simulink model "sim_switch_vol_hover_rotation"  (R2020b)
settings: Solver=VariableStepAuto  StartTime=0.0  StopTime=T  MaxStep=MaxStep  RelTol=RelTol
values from neighbouring files (symbols this model uses):
  J = drone.INERTIA    [utComputeTrimFlight_fmin_dyn.m]
  T = drone.MASS*drone.G    [utComputeTrimFlight_fmin_dyn.m]
undefined symbols (not defined in the file or in its folder): a, b, controlleur, drone, f_initial, K_complet, K_lin_control, q_d_initial, rule, S_complet, u_eq_hover, u_eq_vol, x0, x_eq_hover, x_eq_vol
libraries: simulink x3, simulink_extras x3, sharedtransform x1
settings Model: Creator=florian  LastModifiedBy=florian

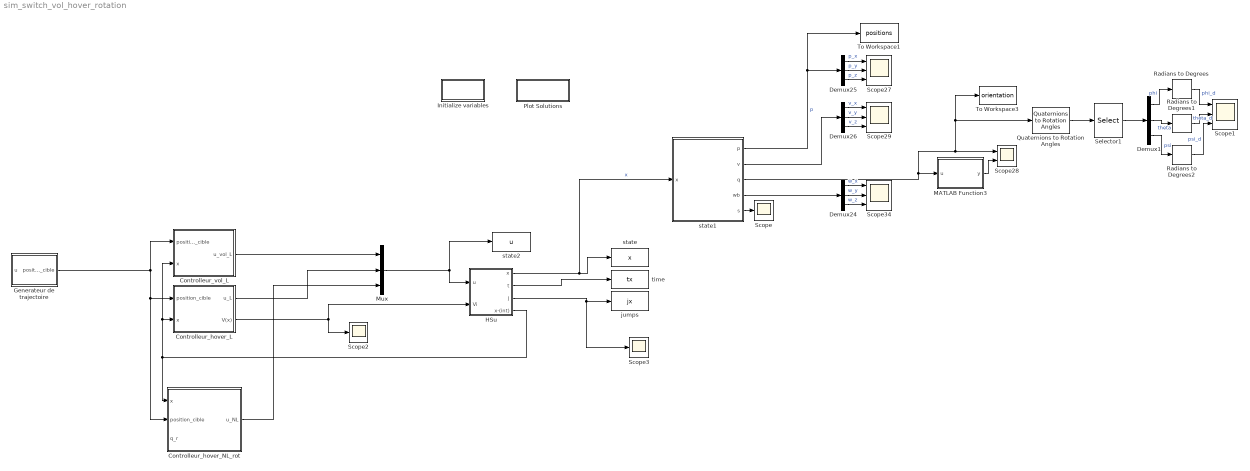
== system sim_switch_vol_hover_rotation ==
  Controlleur_hover_L : Subsystem
  Controlleur_hover_NL_rot : Subsystem
  Controlleur_vol_L : Subsystem
  Demux{1,24..26} (4 alike) : Demux  Outputs=3
  Generateur de trajectoire : MATLAB Function  TreatAsAtomicUnit=on
  HSu : Subsystem  LoadFcn=set_param(gcb,'LinkStatus','none')
      settings: CopyFcn=|
      | set_param(gcb,'LinkStatus','none'),
      | set_param(gcs, 'MaxStep', 'MaxStep', 'RelTol', 'RelTol','Stop time', 'T')
      mask Display:
      | image(imread('Hcal.jpg'))
      | %plot([5 20 20 5 5],[5 5 20 20 5])
      | %text(8,13,'HyEq_mdl')
      | port_label('output', 1, 'x')
      | port_label('output', 2, 't')
      | port_label('output', 3, 'j')
      | port_label('output', 4, 'x-(int)')
      | port_label('input', 1, 'u')
      | port_label('input', 2, 'V(x)')
  Initialize variables : Subsystem  Priority=-10
      settings: OpenFcn=initialization_di
      mask Display: disp('Double Click\n to Initialize')
  MATLAB Function3 : MATLAB Function  TreatAsAtomicUnit=on
  Mux : Mux  Inputs=3
  Plot Solutions : Subsystem
      settings: OpenFcn=postprocessing_di
      mask Display: disp('Double Click to\n Plot Solutions')
  Quaternions to Rotation Angles : sharedtransform/Quaternions to Rotation Angles  rotationOrder=ZXY  aMode=aMode
      settings: SourceProductBaseCode=AE,PW,MT,UV,VE,VP
  Radians to Degrees : simulink_extras/Transformations/Radians to Degrees
  Radians to Degrees1 : simulink_extras/Transformations/Radians to Degrees
  Radians to Degrees2 : simulink_extras/Transformations/Radians to Degrees
  Scope : Scope
  Scope{1,27,29,34} (4 alike) : Scope  NumInputPorts=3
  Scope2 : Scope
  Scope28 : Scope  NumInputPorts=2
  Scope3 : Scope
  Selector1 : Selector  InputPortWidth=3  IndexOptions=Index vector (dialog)  Indices=[2 3 1]  OutputSizes=1
  To Workspace1 : ToWorkspace  VariableName=positions  SampleTime=-1
  To Workspace3 : ToWorkspace  VariableName=orientation  SampleTime=-1
  jumps : ToWorkspace  VariableName=jx  SampleTime=-1
  state : ToWorkspace  VariableName=x  SampleTime=-1
  state1 : MATLAB Function  TreatAsAtomicUnit=on
  state2 : ToWorkspace  VariableName=u  SampleTime=-1
  time : ToWorkspace  VariableName=tx  SampleTime=-1
  wires:
  Mux/1 -> HSu/1(u), state2/1
  HSu/1(x) -> state1/1(x), state/1  "x"
  HSu/2(t) -> time/1
  HSu/3(j) -> jumps/1, Scope3/1
  Controlleur_hover_L/1(u_L) -> Mux/2
  Generateur de trajectoire/1(position_cible) -> Controlleur_vol_L/1(position_cible), Controlleur_hover_NL_rot/2(position_cible), Controlleur_hover_L/1(position_cible)
  Controlleur_hover_L/2(V(x)) -> Scope2/1, HSu/2(Vi)
  HSu/4(x-(int)) -> Controlleur_hover_NL_rot/1(x), Controlleur_vol_L/2(x), Controlleur_hover_L/2(x)
  Demux1/2 -> Radians to Degrees1/1  "theta"
  Quaternions to Rotation Angles/1 -> Selector1/1
  Demux1/3 -> Radians to Degrees2/1  "psi"
  Demux24/2 -> Scope34/2  "w_y"
  Demux26/3 -> Scope29/3  "v_z"
  state1/1(p) -> To Workspace1/1, Demux25/1  "p"
  Demux25/3 -> Scope27/3  "p_z"
  Demux1/1 -> Radians to Degrees/1  "phi"
  Demux25/1 -> Scope27/1  "p_x"
  state1/3(q) -> Scope28/1, To Workspace3/1, Quaternions to Rotation Angles/1, MATLAB Function3/1(u)
  Selector1/1 -> Demux1/1
  Radians to Degrees/1 -> Scope1/1  "phi_d"
  Radians to Degrees1/1 -> Scope1/2  "theta_d"
  Radians to Degrees2/1 -> Scope1/3  "psi_d"
  MATLAB Function3/1(y) -> Scope28/2
  state1/2(v) -> Demux26/1
  Demux26/2 -> Scope29/2  "v_y"
  Demux24/3 -> Scope34/3  "w_z"
  state1/4(wb) -> Demux24/1
  Demux24/1 -> Scope34/1  "w_x"
  Demux26/1 -> Scope29/1  "v_x"
  Demux25/2 -> Scope27/2  "p_y"
  state1/5(s) -> Scope/1
  Controlleur_vol_L/1(u_vol_L) -> Mux/1
  Controlleur_hover_NL_rot/1(u_NL) -> Mux/3

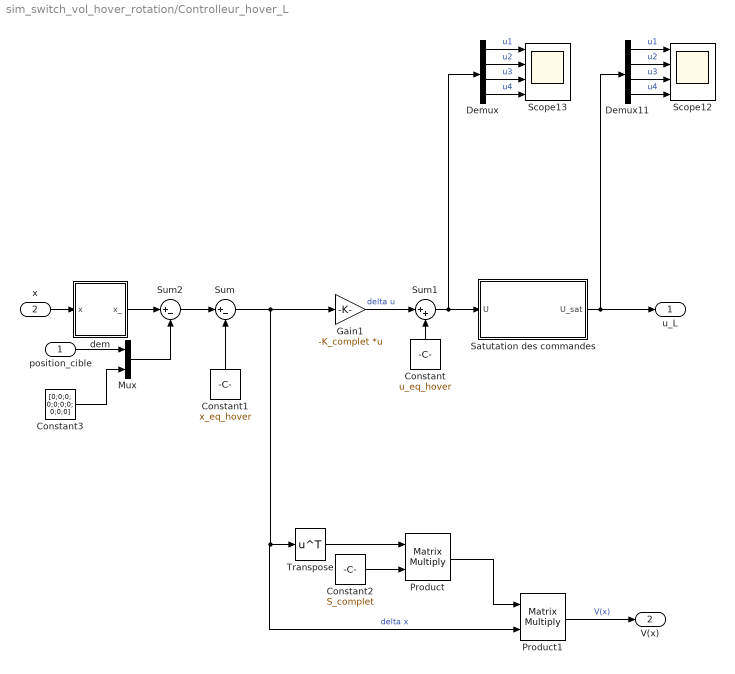
== system sim_switch_vol_hover_rotation/Controlleur_hover_L ==
  position_cible : Inport
  x : Inport  Port=2
  Constant : Constant  Value=u_eq_hover
  Constant1 : Constant  Value=x_eq_hover
  Constant2 : Constant  Value=S_complet
  Constant3 : Constant  Value=[0;0;0; 0;0;0;0; 0;0;0]
  Demux : Demux
  Demux11 : Demux
  Gain1 : Gain  Gain=-K_complet  Multiplication=Matrix(K*u) (u vector)
  Mux : Mux  Inputs=2
  Product : Product  Multiplication=Matrix(*)
  Product1 : Product  Multiplication=Matrix(*)
  Satutation des commandes : Subsystem
  Scope12 : Scope  NumInputPorts=4
  Scope13 : Scope  NumInputPorts=4
  Sum : Sum  Inputs=|+-
  Sum1 : Sum  Inputs=|++
  Sum2 : Sum  Inputs=|+-
  Transpose : Math  Operator=transpose  SaturateOnIntegerOverflow=on
  dem : MATLAB Function  TreatAsAtomicUnit=on
  u_L : Outport
  V(x) : Outport  Port=2
  wires:
  Demux/1 -> Scope13/1  "u1"
  Demux/3 -> Scope13/3  "u3"
  Gain1/1 -> Sum1/1  "delta u"
  Sum1/1 -> Satutation des commandes/1(U), Demux/1
  Sum/1 -> Gain1/1, Product1/2, Transpose/1  "delta x"
  Demux11/3 -> Scope12/3  "u3"
  Satutation des commandes/1(U_sat) -> u_L/1, Demux11/1
  Demux11/2 -> Scope12/2  "u2"
  Product1/1 -> V(x)/1  "V(x)"
  Demux/4 -> Scope13/4  "u4"
  Constant1/1 -> Sum/2
  Transpose/1 -> Product/1
  Product/1 -> Product1/1
  Constant/1 -> Sum1/2
  Demux11/4 -> Scope12/4  "u4"
  Demux/2 -> Scope13/2  "u2"
  Constant2/1 -> Product/2
  Sum2/1 -> Sum/1
  Demux11/1 -> Scope12/1  "u1"
  Mux/1 -> Sum2/2
  position_cible/1 -> Mux/1
  Constant3/1 -> Mux/2
  x/1 -> dem/1(x)
  dem/1(x_) -> Sum2/1

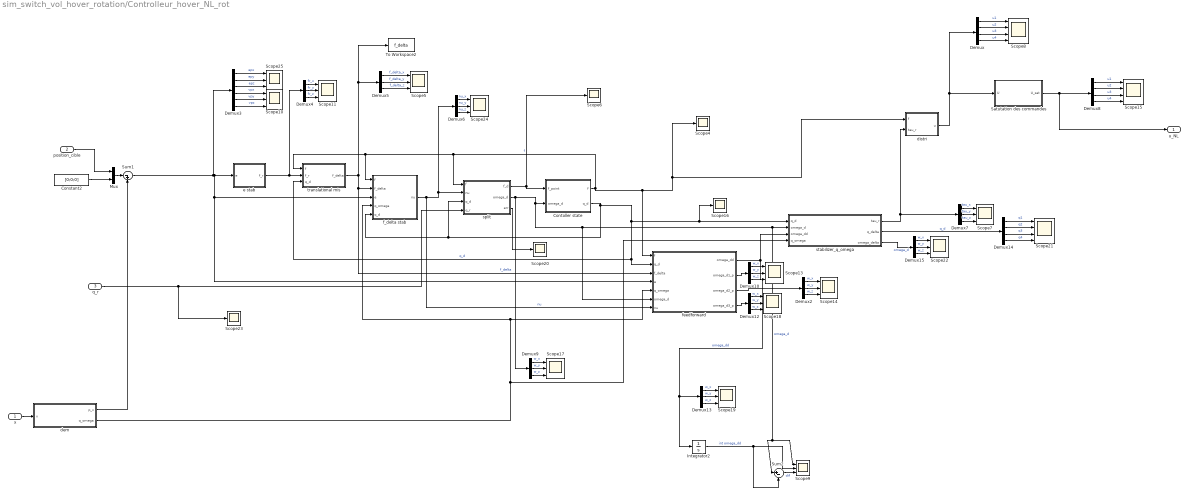
== system sim_switch_vol_hover_rotation/Controlleur_hover_NL_rot ==
  x : Inport
  position_cible : Inport  Port=2
  q_r : Inport  Port=3
  Constant2 : Constant  Value=[0;0;0]
  Contoller state : Subsystem
  Demux : Demux
  Demux{2,4..7,9..10,12..13,15} (10 alike) : Demux  Outputs=3
  Demux14 : Demux
  Demux3 : Demux  Outputs=6
  Demux8 : Demux
  Integrator2 : Integrator
  Mux : Mux  Inputs=2
  Satutation des commandes : Subsystem
  Scope{5,7,9..11,13..14,17..19,22,24..25} (13 alike) : Scope  NumInputPorts=3
  Scope15 : Scope  NumInputPorts=4
  Scope{4,6,16,20,23} (5 alike) : Scope
  Scope21 : Scope  NumInputPorts=4
  Scope8 : Scope  NumInputPorts=4
  Sum1 : Sum  Inputs=|-+
  Sum2 : Sum  Inputs=|+-
  To Workspace2 : ToWorkspace  VariableName=f_delta  SampleTime=-1
  dem : MATLAB Function  TreatAsAtomicUnit=on
  distri : MATLAB Function  TreatAsAtomicUnit=on
  e stab : MATLAB Function  TreatAsAtomicUnit=on
  f_delta stab : MATLAB Function  TreatAsAtomicUnit=on
  feedforward : MATLAB Function  TreatAsAtomicUnit=on
  split : MATLAB Function  TreatAsAtomicUnit=on
  stabilizer_q_omega : MATLAB Function  TreatAsAtomicUnit=on
  translational mis : MATLAB Function  TreatAsAtomicUnit=on
  u_NL : Outport
  wires:
  Demux3/3 -> Scope25/3  "epz"
  Demux15/2 -> Scope22/2  "w_y"
  feedforward/1(omega_dd) -> stabilizer_q_omega/3(omega_dd), Demux13/1, Integrator2/1  "omega_dd"
  split/2(omega_d) -> Demux9/1, feedforward/6(omega_d), Sum2/1, Scope9/1, stabilizer_q_omega/2(omega_d), Contoller state/2(omega_d)  "omega_d"
  Demux3/2 -> Scope25/2  "epy"
  Demux8/4 -> Scope15/4  "u4"
  Demux6/1 -> Scope24/1  "nu_x"
  translational mis/1(f_delta) -> Demux5/1, To Workspace2/1, feedforward/3(f_delta), f_delta stab/2(f_delta)  "f_delta"
  Demux7/2 -> Scope7/2  "tau_y"
  feedforward/3(omega_d2_p) -> Demux2/1
  Demux3/1 -> Scope25/1  "epx"
  Demux8/3 -> Scope15/3  "u3"
  Constant2/1 -> Mux/2
  Demux7/3 -> Scope7/3  "tau_z"
  Demux/3 -> Scope8/3  "u3"
  Demux10/1 -> Scope13/1  "w_x"
  position_cible/1 -> Mux/1
  Demux7/1 -> Scope7/1  "tau_x"
  Satutation des commandes/1(U_sat) -> u_NL/1, Demux8/1
  Demux13/2 -> Scope19/2  "w_y"
  Sum1/1 -> Demux3/1, feedforward/4(e), f_delta stab/3(e), e stab/1(e)
  Demux4/1 -> Scope11/1  "fr_x"
  Demux5/3 -> Scope5/3  "f_delta_z"
  Demux14/1 -> Scope21/1  "q1"
  e stab/1(f_r) -> Demux4/1, translational mis/2(f_r)
  f_delta stab/1(nu) -> feedforward/7(nu), Demux6/1, split/2(nu)  "nu"
  Demux12/2 -> Scope18/2  "w_y"
  q_r/1 -> split/4(q_r), Scope23/1
  Demux6/3 -> Scope24/3  "nu_z"
  Demux8/1 -> Scope15/1  "u1"
  Demux10/2 -> Scope13/2  "w_y"
  Demux9/1 -> Scope17/1  "w_x"
  Mux/1 -> Sum1/1
  Demux12/1 -> Scope18/1  "w_x"
  feedforward/4(omega_d3_p) -> Demux12/1
  Demux/4 -> Scope8/4  "u4"
  Demux8/2 -> Scope15/2  "u2"
  Demux15/1 -> Scope22/1  "w_x"
  Demux5/2 -> Scope5/2  "f_delta_y"
  Demux10/3 -> Scope13/3  "w_z"
  Integrator2/1 -> Sum2/2, Scope9/2  "int omega_dd"
  Demux15/3 -> Scope22/3  "w_z"
  Demux9/2 -> Scope17/2  "w_y"
  Demux2/2 -> Scope14/2  "w_y"
  Demux2/3 -> Scope14/3  "w_z"
  dem/2(q_omega) -> stabilizer_q_omega/4(q_omega), feedforward/5(q_omega), f_delta stab/4(q_omega)
  Demux12/3 -> Scope18/3  "w_z"
  Contoller state/1(f) -> f_delta stab/1(f), translational mis/1(f), split/1(f), feedforward/1(f), Scope4/1, distri/1(f)  "f"
  Demux6/2 -> Scope24/2  "nu_y"
  split/1(f_d) -> Scope6/1, Contoller state/1(f_point)
  Demux/2 -> Scope8/2  "u2"
  Demux13/3 -> Scope19/3  "w_z"
  Demux9/3 -> Scope17/3  "w_z"
  Demux3/4 -> Scope10/1  "vpx"
  Demux2/1 -> Scope14/1  "w_x"
  Demux4/3 -> Scope11/3  "fr_z"
  Contoller state/2(q_d) -> f_delta stab/5(q_d), split/3(q_d), feedforward/2(q_d), translational mis/3(q_d), Scope16/1, stabilizer_q_omega/1(q_d)  "q_d"
  Demux13/1 -> Scope19/1  "w_x"
  Demux3/5 -> Scope10/2  "vpy"
  Demux5/1 -> Scope5/1  "f_delta_x"
  Demux3/6 -> Scope10/3  "vpz"
  Sum2/1 -> Scope9/3  "dif"
  Demux14/2 -> Scope21/2  "q2"
  dem/1(p_v) -> Sum1/2
  Demux4/2 -> Scope11/2  "fr_y"
  stabilizer_q_omega/2(q_delta) -> Demux14/1  "q_d"
  split/3(err) -> Scope20/1
  Demux14/4 -> Scope21/4  "q4"
  Demux/1 -> Scope8/1  "u1"
  stabilizer_q_omega/1(tau_r) -> distri/2(tau_r), Demux7/1
  feedforward/2(omega_d1_p) -> Demux10/1
  stabilizer_q_omega/3(omega_delta) -> Demux15/1  "omega_d"
  distri/1(u) -> Satutation des commandes/1(U), Demux/1
  Demux14/3 -> Scope21/3  "q3"
  x/1 -> dem/1(x)

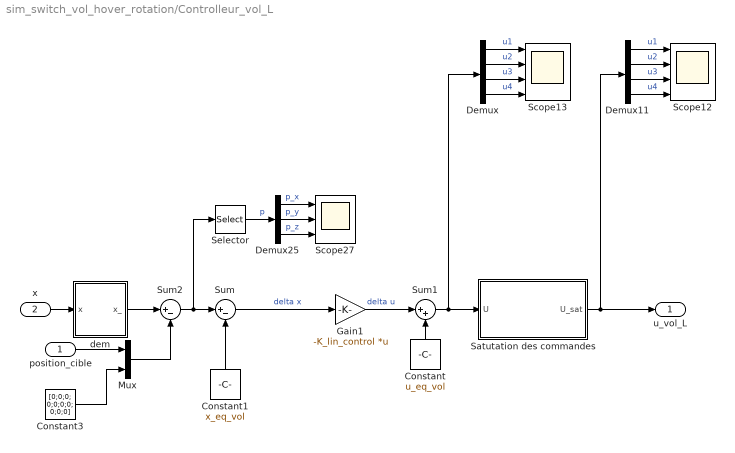
== system sim_switch_vol_hover_rotation/Controlleur_vol_L ==
  position_cible : Inport
  x : Inport  Port=2
  Constant : Constant  Value=u_eq_vol
  Constant1 : Constant  Value=x_eq_vol
  Constant3 : Constant  Value=[0;0;0; 0;0;0;0; 0;0;0]
  Demux : Demux
  Demux11 : Demux
  Demux25 : Demux  Outputs=3
  Gain1 : Gain  Gain=-K_lin_control  Multiplication=Matrix(K*u) (u vector)
  Mux : Mux  Inputs=2
  Satutation des commandes : Subsystem
  Scope12 : Scope  NumInputPorts=4
  Scope13 : Scope  NumInputPorts=4
  Scope27 : Scope  NumInputPorts=3
  Selector : Selector  InputPortWidth=13  IndexOptions=Index vector (dialog)  Indices=[1 2 3]  OutputSizes=1
  Sum : Sum  Inputs=|+-
  Sum1 : Sum  Inputs=|++
  Sum2 : Sum  Inputs=|+-
  dem : MATLAB Function  TreatAsAtomicUnit=on
  u_vol_L : Outport
  wires:
  Demux/1 -> Scope13/1  "u1"
  Demux/3 -> Scope13/3  "u3"
  Gain1/1 -> Sum1/1  "delta u"
  Sum1/1 -> Satutation des commandes/1(U), Demux/1
  Sum/1 -> Gain1/1  "delta x"
  Demux11/3 -> Scope12/3  "u3"
  Satutation des commandes/1(U_sat) -> u_vol_L/1, Demux11/1
  Demux11/2 -> Scope12/2  "u2"
  Demux/4 -> Scope13/4  "u4"
  Constant1/1 -> Sum/2
  Constant/1 -> Sum1/2
  Demux11/4 -> Scope12/4  "u4"
  Demux/2 -> Scope13/2  "u2"
  Sum2/1 -> Selector/1, Sum/1
  Demux11/1 -> Scope12/1  "u1"
  Mux/1 -> Sum2/2
  position_cible/1 -> Mux/1
  Constant3/1 -> Mux/2
  x/1 -> dem/1(x)
  dem/1(x_) -> Sum2/1
  Demux25/3 -> Scope27/3  "p_z"
  Demux25/1 -> Scope27/1  "p_x"
  Selector/1 -> Demux25/1  "p"
  Demux25/2 -> Scope27/2  "p_y"

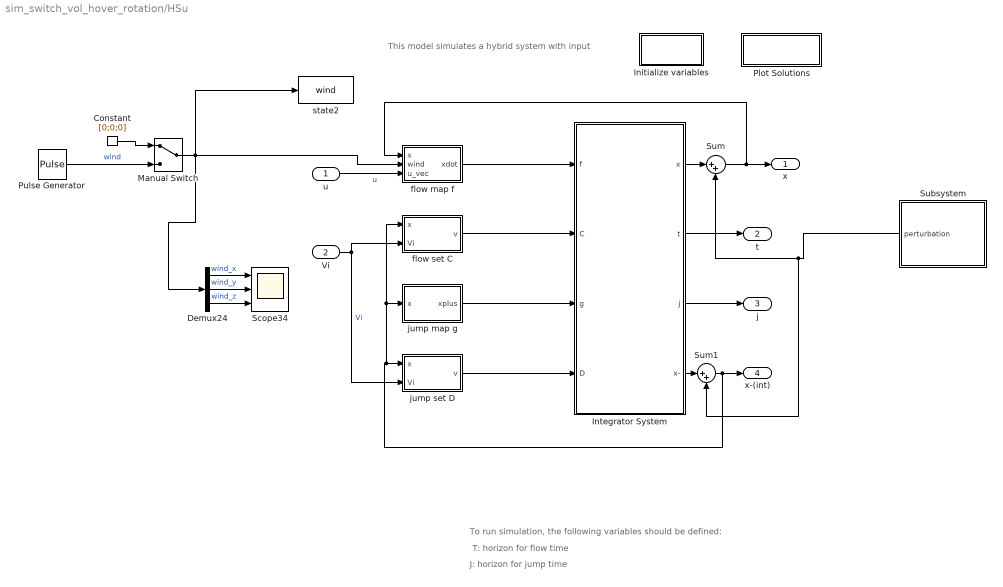
== system sim_switch_vol_hover_rotation/HSu ==
  note: J: horizon for jump time
  note: T: horizon for flow time
  note: To run simulation, the following variables should be defined:
  note: This model simulates a hybrid system with input
  u : Inport
  Vi : Inport  Port=2
  Constant : Constant  Value=[0;0;0]
  Demux24 : Demux  Outputs=3
  Initialize variables : Subsystem  Priority=-10
      settings: OpenFcn=|
      | try
      |      clearvars -except inifile pathfile_in pathfile_pos posfile
      |      cd(pathfile_in);
      |      eval(inifile);
      | catch
      |      [inifile,pathfile_in] = getInitializationfile;
      |      cd(pathfile_in);
      |      inifile = strrep(inifile,'.m','');
      |      eval(inifile);
      | end
      mask Display: disp('Double Click\n to Initialize')
  Integrator System : Subsystem  Priority=2  mask(Hybrid Integrator){T=T, J=J, x0=x0}
      mask prompts: T "Flow Horizon"; J "Jump Horizon"; x0 "Initial Condition"
      mask help:
      | This block integrates the state of the hybrid system defined by the flow map f (first input), the flow set C (second input), the jump map g (third input) and the jump set D (fourth input).
      | Starting from the initial condition x0 (last mask parameter), the system's state x evolves continuously within the set C, according to f(x,u), but is also subject to jumps within D, according to g(x,u).
      | The block also stops the simulation when the time t is greater than the flow horizon T (first mask parameter), or when the number of jumps j is greater than the jump horizon J (second mask parameter).
      | The outputs of the blocks are respectively x(t), t, j, x(t-).
      mask Help:
      | This block integrates the state of the hybrid system defined by the flow map f (first input), the flow set C (second input), the jump map g (third input) and the jump set D (fourth input).
      | <br>
      | Starting from the initial condition x0 (last mask parameter), the system's state x evolves continuously within the set C, according to f(x,u), but is also subject to jumps within D, according to g(x,u).
      | <br>
      | The block also stops the simulation when the time t is greater than the flow horizon T (first mask parameter), or when the number of jumps j is greater than the jump horizon J (second mask parameter).
      | <br>
      | The outputs of the blocks are respectively x(t), t, j, x(t-).
      | <br>
      | You can right click on the block and "Look under mask" to see what's inside the block.
      | Finally, refer to the manual (HybridSimulator_vXX.pdf) for more detailed information on how this hybrid simulator works.
  Manual Switch : ManualSwitch
  Plot Solutions : Subsystem
      settings: OpenFcn=|
      | try
      |      cd(pathfile_pos);
      |      eval(posfile);
      | catch
      |      [posfile,pathfile_pos] = getInitializationfile;
      |      cd(pathfile_pos);
      |      posfile = strrep(posfile,'.m','');
      |      eval(posfile);
      | end
      mask Display: disp('Double Click to\n Plot Solutions')
  Pulse Generator : DiscretePulseGenerator  PulseType=Time based  Amplitude=1.9  Period=10  PulseWidth=30  PhaseDelay=5
  Scope34 : Scope  NumInputPorts=3
  Subsystem : Subsystem
  Sum : Sum  Inputs=|++
  Sum1 : Sum  Inputs=|++
  flow map f : MATLAB Function  TreatAsAtomicUnit=on
  flow set C : MATLAB Function  TreatAsAtomicUnit=on
  jump map g : MATLAB Function  Priority=2  TreatAsAtomicUnit=on
  jump set D : MATLAB Function  TreatAsAtomicUnit=on
  state2 : ToWorkspace  VariableName=wind  SampleTime=-1
  x : Outport
  t : Outport  Port=2
  j : Outport  Port=3
  x-(int) : Outport  Port=4
  wires:
  jump map g/1(xplus) -> Integrator System/3(g)
  jump set D/1(v) -> Integrator System/4(D)
  u/1 -> flow map f/3(u_vec)  "u"
  Integrator System/3(j) -> j/1
  Integrator System/2(t) -> t/1
  flow set C/1(v) -> Integrator System/2(C)
  flow map f/1(xdot) -> Integrator System/1(f)
  Vi/1 -> jump set D/2(Vi), flow set C/2(Vi)  "Vi"
  Constant/1 -> Manual Switch/1
  Manual Switch/1 -> Demux24/1, state2/1, flow map f/2(wind)
  Demux24/1 -> Scope34/1  "wind_x"
  Demux24/2 -> Scope34/2  "wind_y"
  Demux24/3 -> Scope34/3  "wind_z"
  Pulse Generator/1 -> Manual Switch/2  "wind"
  Sum1/1 -> flow set C/1(x), jump map g/1(x), jump set D/1(x), x-(int)/1
  Subsystem/1(perturbation) -> Sum/2, Sum1/2
  Integrator System/1(x) -> Sum/1
  Sum/1 -> flow map f/1(x), x/1
  Integrator System/4(x-) -> Sum1/1

== system sim_switch_vol_hover_rotation/Initialize variables ==

== system sim_switch_vol_hover_rotation/Plot Solutions ==

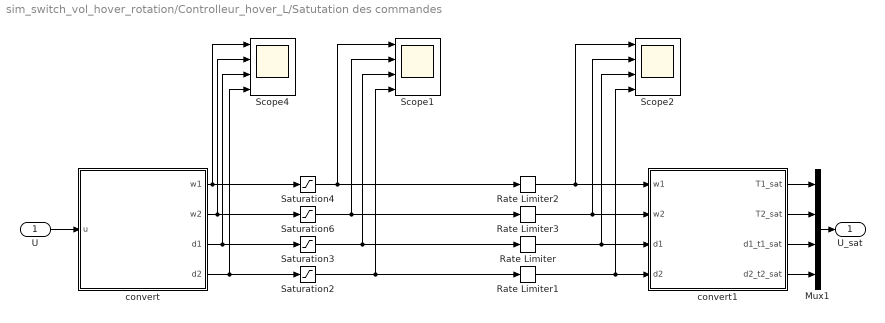
== system sim_switch_vol_hover_rotation/Controlleur_hover_L/Satutation des commandes ==
  U : Inport
  Mux1 : Mux
  Rate Limiter : RateLimiter  RisingSlewLimit=drone.ELEVON_RATE_CHANGE  FallingSlewLimit=-drone.ELEVON_RATE_CHANGE  SampleTimeMode=inherited
  Rate Limiter1 : RateLimiter  RisingSlewLimit=drone.ELEVON_RATE_CHANGE  FallingSlewLimit=-drone.ELEVON_RATE_CHANGE  SampleTimeMode=inherited
  Rate Limiter2 : RateLimiter  RisingSlewLimit=drone.MOTOR_RATE_CHANGE  FallingSlewLimit=-drone.MOTOR_RATE_CHANGE  SampleTimeMode=inherited
  Rate Limiter3 : RateLimiter  RisingSlewLimit=drone.MOTOR_RATE_CHANGE  FallingSlewLimit=-drone.MOTOR_RATE_CHANGE  SampleTimeMode=inherited
  Saturation2 : Saturate  UpperLimit=30*(pi/180)  LowerLimit=-30*(pi/180)
  Saturation3 : Saturate  UpperLimit=30*(pi/180)  LowerLimit=-30*(pi/180)
  Saturation4 : Saturate  UpperLimit=1000  LowerLimit=200
  Saturation6 : Saturate  UpperLimit=1000  LowerLimit=200
  Scope1 : Scope  NumInputPorts=4
  Scope2 : Scope  NumInputPorts=4
  Scope4 : Scope  NumInputPorts=4
  convert : MATLAB Function  TreatAsAtomicUnit=on
  convert1 : MATLAB Function  TreatAsAtomicUnit=on
  U_sat : Outport
  wires:
  convert/1(w1) -> Saturation4/1, Scope4/1
  Saturation3/1 -> Rate Limiter/1, Scope1/3
  convert/2(w2) -> Scope4/2, Saturation6/1
  convert/3(d1) -> Scope4/3, Saturation3/1
  convert/4(d2) -> Saturation2/1, Scope4/4
  convert1/1(T1_sat) -> Mux1/1
  convert1/4(d2_t2_sat) -> Mux1/4
  Mux1/1 -> U_sat/1
  convert1/2(T2_sat) -> Mux1/2
  convert1/3(d1_t1_sat) -> Mux1/3
  Saturation2/1 -> Rate Limiter1/1, Scope1/4
  Rate Limiter/1 -> Scope2/3, convert1/3(d1)
  Saturation6/1 -> Rate Limiter3/1, Scope1/2
  Saturation4/1 -> Rate Limiter2/1, Scope1/1
  Rate Limiter1/1 -> Scope2/4, convert1/4(d2)
  Rate Limiter2/1 -> Scope2/1, convert1/1(w1)
  Rate Limiter3/1 -> Scope2/2, convert1/2(w2)
  U/1 -> convert/1(u)

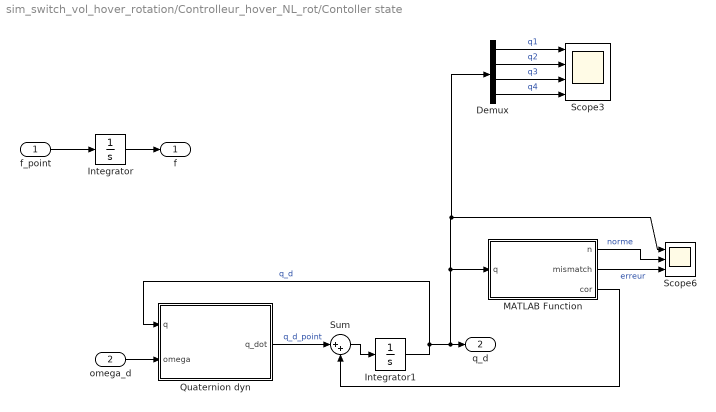
== system sim_switch_vol_hover_rotation/Controlleur_hover_NL_rot/Contoller state ==
  f_point : Inport
  omega_d : Inport  Port=2
  Demux : Demux
  Integrator : Integrator  InitialCondition=f_initial
  Integrator1 : Integrator  InitialCondition=q_d_initial
  MATLAB Function : MATLAB Function  TreatAsAtomicUnit=on
  Quaternion dyn : MATLAB Function  TreatAsAtomicUnit=on
  Scope3 : Scope  NumInputPorts=4
  Scope6 : Scope  NumInputPorts=3
  Sum : Sum  Inputs=|++
  f : Outport
  q_d : Outport  Port=2
  wires:
  Integrator/1 -> f/1
  f_point/1 -> Integrator/1
  Integrator1/1 -> Quaternion dyn/1(q), Demux/1, Scope6/1, MATLAB Function/1(q), q_d/1  "q_d"
  omega_d/1 -> Quaternion dyn/2(omega)
  Quaternion dyn/1(q_dot) -> Sum/1  "q_d_point"
  Sum/1 -> Integrator1/1
  MATLAB Function/3(cor) -> Sum/2
  MATLAB Function/1(n) -> Scope6/2  "norme"
  MATLAB Function/2(mismatch) -> Scope6/3  "erreur"
  Demux/3 -> Scope3/3  "q3"
  Demux/2 -> Scope3/2  "q2"
  Demux/1 -> Scope3/1  "q1"
  Demux/4 -> Scope3/4  "q4"

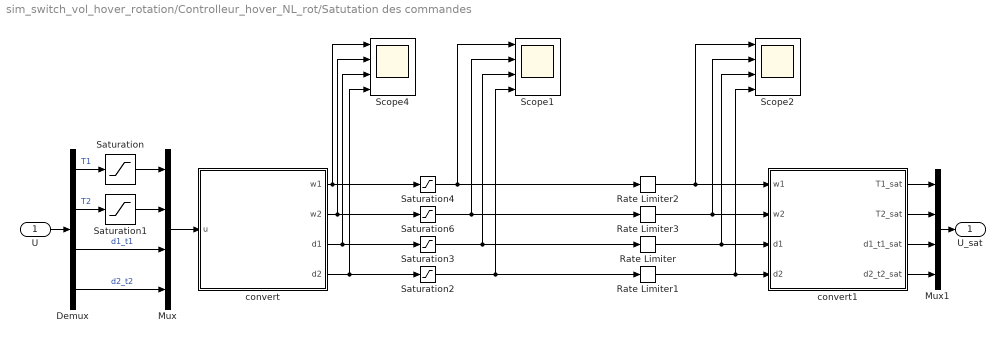
== system sim_switch_vol_hover_rotation/Controlleur_hover_NL_rot/Satutation des commandes ==
  U : Inport
  Demux : Demux
  Mux : Mux
  Mux1 : Mux
  Rate Limiter : RateLimiter  RisingSlewLimit=drone.ELEVON_RATE_CHANGE  FallingSlewLimit=-drone.ELEVON_RATE_CHANGE  SampleTimeMode=inherited
  Rate Limiter1 : RateLimiter  RisingSlewLimit=drone.ELEVON_RATE_CHANGE  FallingSlewLimit=-drone.ELEVON_RATE_CHANGE  SampleTimeMode=inherited
  Rate Limiter2 : RateLimiter  RisingSlewLimit=drone.MOTOR_RATE_CHANGE  FallingSlewLimit=-drone.MOTOR_RATE_CHANGE  SampleTimeMode=inherited
  Rate Limiter3 : RateLimiter  RisingSlewLimit=drone.MOTOR_RATE_CHANGE  FallingSlewLimit=-drone.MOTOR_RATE_CHANGE  SampleTimeMode=inherited
  Saturation : Saturate  UpperLimit=100  LowerLimit=0.001
  Saturation1 : Saturate  UpperLimit=100  LowerLimit=0.001
  Saturation2 : Saturate  UpperLimit=30*(pi/180)  LowerLimit=-30*(pi/180)
  Saturation3 : Saturate  UpperLimit=30*(pi/180)  LowerLimit=-30*(pi/180)
  Saturation4 : Saturate  UpperLimit=1000  LowerLimit=200
  Saturation6 : Saturate  UpperLimit=1000  LowerLimit=200
  Scope1 : Scope  NumInputPorts=4
  Scope2 : Scope  NumInputPorts=4
  Scope4 : Scope  NumInputPorts=4
  convert : MATLAB Function  TreatAsAtomicUnit=on
  convert1 : MATLAB Function  TreatAsAtomicUnit=on
  U_sat : Outport
  wires:
  U/1 -> Demux/1
  Demux/4 -> Mux/4  "d2_t2"
  Demux/1 -> Saturation/1  "T1"
  Demux/3 -> Mux/3  "d1_t1"
  Demux/2 -> Saturation1/1  "T2"
  Saturation/1 -> Mux/1
  Mux/1 -> convert/1(u)
  convert/1(w1) -> Saturation4/1, Scope4/1
  Saturation3/1 -> Rate Limiter/1, Scope1/3
  convert/2(w2) -> Scope4/2, Saturation6/1
  convert/3(d1) -> Scope4/3, Saturation3/1
  convert/4(d2) -> Saturation2/1, Scope4/4
  convert1/1(T1_sat) -> Mux1/1
  convert1/4(d2_t2_sat) -> Mux1/4
  Mux1/1 -> U_sat/1
  Saturation1/1 -> Mux/2
  convert1/2(T2_sat) -> Mux1/2
  convert1/3(d1_t1_sat) -> Mux1/3
  Saturation2/1 -> Rate Limiter1/1, Scope1/4
  Rate Limiter/1 -> Scope2/3, convert1/3(d1)
  Saturation6/1 -> Rate Limiter3/1, Scope1/2
  Saturation4/1 -> Rate Limiter2/1, Scope1/1
  Rate Limiter1/1 -> Scope2/4, convert1/4(d2)
  Rate Limiter2/1 -> Scope2/1, convert1/1(w1)
  Rate Limiter3/1 -> Scope2/2, convert1/2(w2)

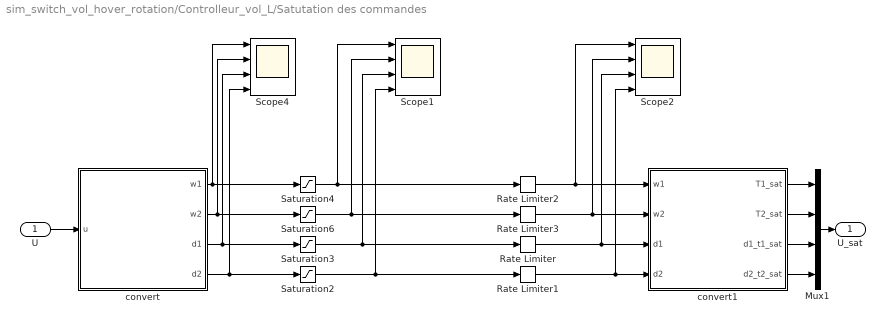
== system sim_switch_vol_hover_rotation/Controlleur_vol_L/Satutation des commandes ==
  U : Inport
  Mux1 : Mux
  Rate Limiter : RateLimiter  RisingSlewLimit=drone.ELEVON_RATE_CHANGE  FallingSlewLimit=-drone.ELEVON_RATE_CHANGE  SampleTimeMode=inherited
  Rate Limiter1 : RateLimiter  RisingSlewLimit=drone.ELEVON_RATE_CHANGE  FallingSlewLimit=-drone.ELEVON_RATE_CHANGE  SampleTimeMode=inherited
  Rate Limiter2 : RateLimiter  RisingSlewLimit=drone.MOTOR_RATE_CHANGE  FallingSlewLimit=-drone.MOTOR_RATE_CHANGE  SampleTimeMode=inherited
  Rate Limiter3 : RateLimiter  RisingSlewLimit=drone.MOTOR_RATE_CHANGE  FallingSlewLimit=-drone.MOTOR_RATE_CHANGE  SampleTimeMode=inherited
  Saturation2 : Saturate  UpperLimit=30*(pi/180)  LowerLimit=-30*(pi/180)
  Saturation3 : Saturate  UpperLimit=30*(pi/180)  LowerLimit=-30*(pi/180)
  Saturation4 : Saturate  UpperLimit=1000  LowerLimit=200
  Saturation6 : Saturate  UpperLimit=1000  LowerLimit=200
  Scope1 : Scope  NumInputPorts=4
  Scope2 : Scope  NumInputPorts=4
  Scope4 : Scope  NumInputPorts=4
  convert : MATLAB Function  TreatAsAtomicUnit=on
  convert1 : MATLAB Function  TreatAsAtomicUnit=on
  U_sat : Outport
  wires:
  convert/1(w1) -> Saturation4/1, Scope4/1
  Saturation3/1 -> Rate Limiter/1, Scope1/3
  convert/2(w2) -> Scope4/2, Saturation6/1
  convert/3(d1) -> Scope4/3, Saturation3/1
  convert/4(d2) -> Saturation2/1, Scope4/4
  convert1/1(T1_sat) -> Mux1/1
  convert1/4(d2_t2_sat) -> Mux1/4
  Mux1/1 -> U_sat/1
  convert1/2(T2_sat) -> Mux1/2
  convert1/3(d1_t1_sat) -> Mux1/3
  Saturation2/1 -> Rate Limiter1/1, Scope1/4
  Rate Limiter/1 -> Scope2/3, convert1/3(d1)
  Saturation6/1 -> Rate Limiter3/1, Scope1/2
  Saturation4/1 -> Rate Limiter2/1, Scope1/1
  Rate Limiter1/1 -> Scope2/4, convert1/4(d2)
  Rate Limiter2/1 -> Scope2/1, convert1/1(w1)
  Rate Limiter3/1 -> Scope2/2, convert1/2(w2)
  U/1 -> convert/1(u)

== system sim_switch_vol_hover_rotation/HSu/Initialize variables ==

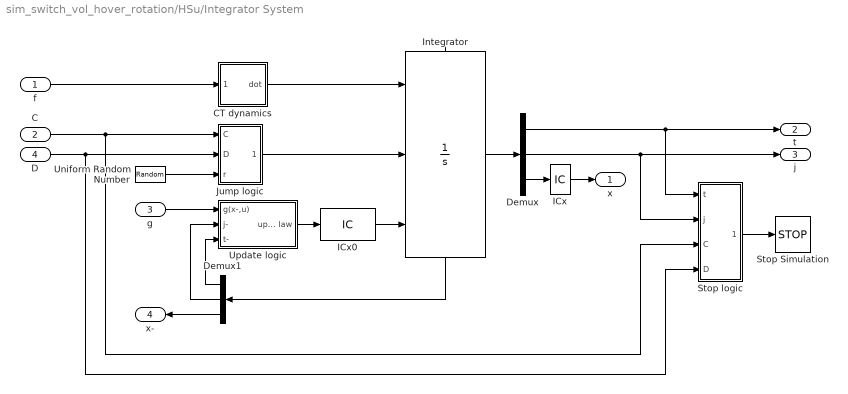
== system sim_switch_vol_hover_rotation/HSu/Integrator System ==
  f : Inport
  C : Inport  Port=2
  g : Inport  Port=3
  D : Inport  Port=4
  CT dynamics : Subsystem
  Demux : Demux  Outputs=[1 1 -1]
  Demux1 : Demux  Outputs=[1 1 -1]
  ICx : InitialCondition  Value=x0
  ICx0 : InitialCondition  Value=[0; 0; x0(:)]
  Integrator : Integrator  ExternalReset=level hold  InitialConditionSource=external  ShowStatePort=on  ZeroCross=off
  Jump logic : Subsystem
  Stop Simulation : Stop
  Stop logic : Subsystem
  Uniform Random Number : UniformRandomNumber  Minimum=0  Seed=abs(floor(100*rand))  SampleTime=0
  Update logic : Subsystem
  x : Outport
  t : Outport  Port=2
  j : Outport  Port=3
  x- : Outport  Port=4
  wires:
  ICx0/1 -> Integrator/3
  ICx/1 -> x/1
  Demux/3 -> ICx/1
  Integrator/State -> Demux1/1
  Demux/2 -> j/1, Stop logic/2(j)
  Demux/1 -> t/1, Stop logic/1(t)
  Update logic/1(update law) -> ICx0/1
  CT dynamics/1(dot) -> Integrator/1
  Stop logic/1(stop) -> Stop Simulation/1
  Integrator/1 -> Demux/1
  C/1 -> Stop logic/3(C), Jump logic/1(C)
  D/1 -> Stop logic/4(D), Jump logic/2(D)
  f/1 -> CT dynamics/1(f(x,u))
  Demux1/3 -> x-/1
  Jump logic/1(jump) -> Integrator/2
  Uniform Random Number/1 -> Jump logic/3(r)
  g/1 -> Update logic/1(g(x-,u))
  Demux1/1 -> Update logic/3(t-)
  Demux1/2 -> Update logic/2(j-)

== system sim_switch_vol_hover_rotation/HSu/Plot Solutions ==

== system sim_switch_vol_hover_rotation/HSu/Subsystem ==
  Clock : Clock
  MATLAB Function : MATLAB Function  TreatAsAtomicUnit=on
  perturbation : Outport
  wires:
  Clock/1 -> MATLAB Function/1(t)
  MATLAB Function/1(y) -> perturbation/1

== system sim_switch_vol_hover_rotation/HSu/Integrator System/CT dynamics ==
  f(x,u) : Inport
  Flows : Constant
  Jumps : Constant  Value=0
  Mux : Mux  Inputs=[1 1 -1]
  dot : Outport
  wires:
  Jumps/1 -> Mux/2
  Flows/1 -> Mux/1
  Mux/1 -> dot/1
  f(x,u)/1 -> Mux/3

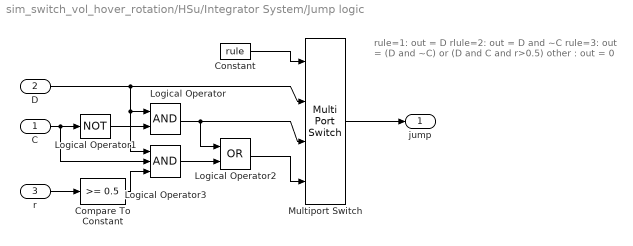
== system sim_switch_vol_hover_rotation/HSu/Integrator System/Jump logic ==
  note: rule=1:  out = D
      | rlule=2: out = D and ~C
      | rule=3:  out = (D and ~C)  or (D and C and r>0.5)
      | other :  out = 0
  C : Inport
  D : Inport  Port=2
  r : Inport  Port=3
  Compare To Constant : simulink/Logic and Bit Operations/Compare To Constant  relop=>=  const=0.5  OutDataTypeStr=uint8
  Constant : Constant  Value=rule
  Logical Operator : Logic  AllPortsSameDT=off  OutDataTypeStr=boolean
  Logical Operator1 : Logic  Operator=NOT  Inputs=1  AllPortsSameDT=off  OutDataTypeStr=boolean
  Logical Operator2 : Logic  Operator=OR  AllPortsSameDT=off  OutDataTypeStr=boolean
  Logical Operator3 : Logic  Inputs=3  AllPortsSameDT=off  OutDataTypeStr=boolean
  Multiport Switch : MultiPortSwitch
  jump : Outport
  wires:
  Constant/1 -> Multiport Switch/1
  D/1 -> Logical Operator3/1, Logical Operator/1, Multiport Switch/2
  r/1 -> Compare To Constant/1
  C/1 -> Logical Operator3/2, Logical Operator1/1
  Logical Operator1/1 -> Logical Operator/2
  Logical Operator/1 -> Multiport Switch/3, Logical Operator2/1
  Logical Operator2/1 -> Multiport Switch/4
  Multiport Switch/1 -> jump/1
  Compare To Constant/1 -> Logical Operator3/3
  Logical Operator3/1 -> Logical Operator2/2

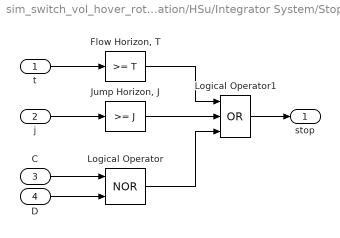
== system sim_switch_vol_hover_rotation/HSu/Integrator System/Stop logic ==
  t : Inport
  j : Inport  Port=2
  C : Inport  Port=3
  D : Inport  Port=4
  "Flow Horizon, T" : simulink/Logic and Bit Operations/Compare To Constant  relop=>=  const=T  OutDataTypeStr=uint8  ZeroCross=off
  "Jump Horizon, J" : simulink/Logic and Bit Operations/Compare To Constant  relop=>=  const=J  OutDataTypeStr=uint8  ZeroCross=off
  Logical Operator : Logic  Operator=NOR  AllPortsSameDT=off  OutDataTypeStr=boolean
  Logical Operator1 : Logic  Operator=OR  Inputs=3  AllPortsSameDT=off  OutDataTypeStr=boolean
  stop : Outport
  wires:
  "Flow Horizon, T"/1 -> Logical Operator1/1
  "Jump Horizon, J"/1 -> Logical Operator1/2
  Logical Operator/1 -> Logical Operator1/3
  D/1 -> Logical Operator/2
  t/1 -> "Flow Horizon, T"/1
  j/1 -> "Jump Horizon, J"/1
  C/1 -> Logical Operator/1
  Logical Operator1/1 -> stop/1

== system sim_switch_vol_hover_rotation/HSu/Integrator System/Update logic ==
  g(x-,u) : Inport
  j- : Inport  Port=2
  t- : Inport  Port=3
  Constant : Constant
  Mux1 : Mux  Inputs=[1 1 -1]
  Sum : Sum  Inputs=|++
  update law : Outport
  wires:
  Sum/1 -> Mux1/2
  Mux1/1 -> update law/1
  j-/1 -> Sum/1
  g(x-,u)/1 -> Mux1/3
  t-/1 -> Mux1/1
  Constant/1 -> Sum/2

== matlab function sim_switch_vol_hover_rotation/Controlleur_hover_NL_rot/Contoller state/MATLAB Function ==
  data: n output; q input; mismatch output; cor output
function [n, mismatch, cor] = fcn(q)
%#codegen
n = norm(q);
mismatch = 1-norm(q);
cor = mismatch*q;

== matlab function sim_switch_vol_hover_rotation/Controlleur_hover_NL_rot/Satutation des commandes/convert ==
  data: u input; w1 output; drone parameter; w2 output; d1 output; d2 output
function [w1, w2, d1, d2] = convert(u, drone)
%#codegen
kf = drone.PROP_KP;

T1 = u(1);
T2 = u(2);
d1_T1 = u(3);
d2_T2 = u(4);

w1 = sqrt(T1/kf);
w2 = sqrt(T2/kf);
d1 = d1_T1/T1;
d2 = d2_T2/T2;

== matlab function sim_switch_vol_hover_rotation/Controlleur_hover_NL_rot/Contoller state/Quaternion dyn ==
  data: q input; q_dot output; omega input
function q_dot = q_dyn(q, omega)
%#codegen

eta = q(1);
eps = q(2:4);

A = [-eps';  eta*eye(3)+skew_sym(eps)];
q_dot = 1/2*A*omega;

== matlab function sim_switch_vol_hover_rotation/Controlleur_hover_NL_rot/Satutation des commandes/convert1 ==
  data: w1 input; w2 input; d1 input; d2 input; T1_sat output; T2_sat output; drone parameter; d1_t1_sat output; d2_t2_sat output
function [T1_sat, T2_sat, d1_t1_sat, d2_t2_sat] = convert2(w1, w2, d1, d2, drone)
%#codegen
kf = drone.PROP_KP;

T1_sat = kf*w1^2;
d1_t1_sat = d1*T1_sat;
T2_sat = kf*w2^2;
d2_t2_sat = d2*T2_sat;

== matlab function sim_switch_vol_hover_rotation/HSu/flow map f ==
  data: x input; wind input; xdot output; u_vec input; drone parameter
function xdot = f(x, wind, u_vec, drone)
%--------------------------------------------------------------------------
% Matlab M-file Project: HyEQ Toolbox @  Hybrid Systems Laboratory (HSL), 
% https://hybrid.soe.ucsc.edu/software
% http://hybridsimulator.wordpress.com/
%--------------------------------------------------------------------------
% Project: Simulation of a hybrid system
% Description: Flow map
%--------------------------------------------------------------------------
%--------------------------------------------------------------------------
%   See also HYEQSOLVER, PLOTARC, PLOTARC3, PLOTFLOWS, PLOTHARC,
%   PLOTHARCCOLOR, PLOTHARCCOLOR3D, PLOTHYBRIDARC, PLOTJUMPS.
%   Copyright @ Hybrid Systems Laboratory (HSL),
%   Revision: 0.0.0.3 Date: 05/20/2015 3:42:00
%--------------------------------------------------------------------------
% flow map: xdot=f(x,u);

%% physical constants
% gravity
g = drone.G;
% vehicle mass
m = drone.MASS;
% vehicle inertia matrix
J = drone.INERTIA; % [3x3 real symmetric] in body axis

%% state demultiplexing
% p = x(1:3);
v = x(4:6);
q  = x(7:10);
wb = x(11:13);
s = x(14);

%% Commande switch s = 0 => contolleur vol L, s = 1 => contolleur hover L , s = 2 => contolleur hover NL rot

if(s == 0)
    u = u_vec(1:4);
elseif(s == 1)
    u = u_vec(5:8);
elseif(s == 2)
    u = u_vec(9:12);
end
    

Rq = q2dcm(q);

[Fp, Mp] = external_force_moment(x, u, wind, drone);

% position
dpdt = v;

% kinematics
dvdt =  -[0;0;g] + (1/m)*Rq*drone.Fb*u + (1/m)*Rq*Fp; 

%% quaternion derivative
eta = q(1);
eps = q(2:4);

dqdt = (1/2)*[-eps'; eta*eye(3) + skew_sym(eps)]*wb;

%% angular velocity derivative
% kinematics
dwdt = -J\cross(wb, J*wb) + J\(drone.Mb*u) + J\Mp;


%% derivative multiplexing
xdot = [dpdt; dvdt; dqdt; dwdt; 0] ;

== matlab function sim_switch_vol_hover_rotation/HSu/flow set C ==
  data: x input; v output; Vi input; a parameter; b parameter
function v   = C(x, Vi, a, b) 
%--------------------------------------------------------------------------
% Matlab M-file Project: HyEQ Toolbox @  Hybrid Systems Laboratory (HSL), 
% https://hybrid.soe.ucsc.edu/software
% http://hybridsimulator.wordpress.com/
%--------------------------------------------------------------------------
% Project: Simulation of a hybrid system
% Description: Flow set
%--------------------------------------------------------------------------
%--------------------------------------------------------------------------
%   See also HYEQSOLVER, PLOTARC, PLOTARC3, PLOTFLOWS, PLOTHARC,
%   PLOTHARCCOLOR, PLOTHARCCOLOR3D, PLOTHYBRIDARC, PLOTJUMPS.
%   Copyright @ Hybrid Systems Laboratory (HSL),
%   Revision: 0.0.0.3 Date: 05/20/2015 3:42:00
%
%state
s = x(14);


if (((Vi <= b ) && (s == 0)) || ((Vi >= a ) && (s == 1)))  % flow condition
    v = 1;  % report flow
else
    v = 0;   % do not report flow
end

== matlab function sim_switch_vol_hover_rotation/HSu/jump map g ==
  data: x input; xplus output
function xplus = g(x)
%--------------------------------------------------------------------------
% Matlab M-file Project: HyEQ Toolbox @  Hybrid Systems Laboratory (HSL), 
% https://hybrid.soe.ucsc.edu/software
% http://hybridsimulator.wordpress.com/
%--------------------------------------------------------------------------
% Project: Simulation of a hybrid system
% Description: Jump map
%--------------------------------------------------------------------------
%--------------------------------------------------------------------------
%   See also HYEQSOLVER, PLOTARC, PLOTARC3, PLOTFLOWS, PLOTHARC,
%   PLOTHARCCOLOR, PLOTHARCCOLOR3D, PLOTHYBRIDARC, PLOTJUMPS.
%   Copyright @ Hybrid Systems Laboratory (HSL),
%   Revision: 0.0.0.3 Date: 05/20/2015 3:42:00
%--------------------------------------------------------------------------

xplus = [x(1:13); 1-x(14)];

== matlab function sim_switch_vol_hover_rotation/HSu/jump set D ==
  data: x input; v output; Vi input; a parameter; b parameter
function v  = D(x, Vi, a, b) 
%--------------------------------------------------------------------------
% Matlab M-file Project: HyEQ Toolbox @  Hybrid Systems Laboratory (HSL), 
% https://hybrid.soe.ucsc.edu/software
% http://hybridsimulator.wordpress.com/
%--------------------------------------------------------------------------
% Project: Simulation of a hybrid system
% Description: Jump set
%--------------------------------------------------------------------------
%--------------------------------------------------------------------------
%   See also HYEQSOLVER, PLOTARC, PLOTARC3, PLOTFLOWS, PLOTHARC,
%   PLOTHARCCOLOR, PLOTHARCCOLOR3D, PLOTHYBRIDARC, PLOTJUMPS.
%   Copyright @ Hybrid Systems Laboratory (HSL),
%   Revision: 0.0.0.3 Date: 05/20/2015 3:42:00
%
%state
s = x(14);

if ( ((Vi >= b ) && (s == 0)) || ((Vi <= a ) && (s == 1)))  % jump condition
    v = 1;  % report jump
else
    v = 0;   % do not report jump
end

== matlab function sim_switch_vol_hover_rotation/Controlleur_hover_NL_rot/translational mis ==
  data: f input; f_r input; f_delta output; q_d input; controlleur parameter
function f_delta = trans_mis(f, f_r,  q_d, controlleur)
%#codegen

f_delta = q2dcm(q_d) * controlleur.d_etoile * f - f_r;

== matlab function sim_switch_vol_hover_rotation/Controlleur_hover_L/dem ==
  data: x input; x_ output
function x_ = demux(x)

x_ = x(1:13);

== matlab function sim_switch_vol_hover_rotation/Controlleur_hover_L/Satutation des commandes/convert ==
  data: u input; w1 output; drone parameter; w2 output; d1 output; d2 output
function [w1, w2, d1, d2] = convert(u, drone)
%#codegen
kf = drone.PROP_KP;

T1 = max(u(1),0);
T2 = max(u(2),0);
d1_T1 = u(3);
d2_T2 = u(4);

w1 = sqrt(T1/kf);
w2 = sqrt(T2/kf);
d1 = d1_T1/T1;
d2 = d2_T2/T2;

== matlab function sim_switch_vol_hover_rotation/Controlleur_hover_L/Satutation des commandes/convert1 ==
  data: w1 input; w2 input; d1 input; d2 input; T1_sat output; T2_sat output; drone parameter; d1_t1_sat output; d2_t2_sat output
function [T1_sat, T2_sat, d1_t1_sat, d2_t2_sat] = convert2(w1, w2, d1, d2, drone)
%#codegen
kf = drone.PROP_KP;

T1_sat = kf*w1^2;
d1_t1_sat = d1*T1_sat;
T2_sat = kf*w2^2;
d2_t2_sat = d2*T2_sat;

== matlab function sim_switch_vol_hover_rotation/HSu/Subsystem/MATLAB Function ==
  data: t input; y output
function y = disturbance(t)
    if(t>10)

%         y = [50; zeros(13,1)];
        y = zeros(14,1);
    else
        y = zeros(14,1);
    end
end

== matlab function sim_switch_vol_hover_rotation/Generateur de trajectoire ==
  data: u input; position_cible output; list_point parameter
function position_cible = traj(u, list_point)
%#codegen

position_cible = 1;

== matlab function sim_switch_vol_hover_rotation/Controlleur_hover_NL_rot/distri ==
  data: f input; u output; tau_r input; controlleur parameter
function u = dist(f,tau_r, controlleur)
%#codegen
u = controlleur.M_k * tau_r + controlleur.u_barre * f;

== matlab function sim_switch_vol_hover_rotation/Controlleur_vol_L/Satutation des commandes/convert ==
  data: u input; w1 output; drone parameter; w2 output; d1 output; d2 output
function [w1, w2, d1, d2] = convert(u, drone)
%#codegen
kf = drone.PROP_KP;

T1 = max(u(1),0);
T2 = max(u(2),0);
d1_T1 = u(3);
d2_T2 = u(4);

w1 = sqrt(T1/kf);
w2 = sqrt(T2/kf);
d1 = d1_T1/T1;
d2 = d2_T2/T2;

== matlab function sim_switch_vol_hover_rotation/state1 ==
  data: x input; p output; v output; q output; wb output; s output
function [p, v,q, wb, s] = demux(x)
%#codegen

p = x(1:3);
v = x(4:6);
q  = x(7:10);
wb = x(11:13);
s = x(14);

== matlab function sim_switch_vol_hover_rotation/Controlleur_vol_L/Satutation des commandes/convert1 ==
  data: w1 input; w2 input; d1 input; d2 input; T1_sat output; T2_sat output; drone parameter; d1_t1_sat output; d2_t2_sat output
function [T1_sat, T2_sat, d1_t1_sat, d2_t2_sat] = convert2(w1, w2, d1, d2, drone)
%#codegen
kf = drone.PROP_KP;

T1_sat = kf*w1^2;
d1_t1_sat = d1*T1_sat;
T2_sat = kf*w2^2;
d2_t2_sat = d2*T2_sat;

== matlab function sim_switch_vol_hover_rotation/Controlleur_vol_L/dem ==
  data: x input; x_ output
function x_ = demux(x)

x_ = x(1:13);

== matlab function sim_switch_vol_hover_rotation/Controlleur_hover_NL_rot/dem ==
  data: x input; p_v output; q_omega output
function [p_v, q_omega] = demux(x)

p_v = x(1:6);
q_omega = x(7:13);

== matlab function sim_switch_vol_hover_rotation/Controlleur_hover_NL_rot/stabilizer_q_omega ==
  data: q_d input; omega_d input; omega_dd input; q_omega input; tau_r output; controlleur parameter; drone parameter; q_delta output; omega_delta output
function [tau_r, q_delta, omega_delta]  = stabilizer_q_omega(q_d, omega_d, omega_dd, q_omega, controlleur, drone )

J = drone.INERTIA;

q = q_omega(1:4);
omega = q_omega(5:7);

eta = q(1);
eps = q(2:4);

eta_d = q_d(1);
eps_d = q_d(2:4);

eta_delta = eta_d*eta + eps_d'*eps;
eps_delta = -eta*eps_d + eta_d*eps - skew_sym(eps_d)*eps;

omega_delta = omega - omega_d;

tau_r = - controlleur.kap * eps_delta - controlleur.kad * omega_delta + cross(omega, J* omega) + J*omega_dd;
q_delta = [eta_delta; eps_delta];
end

== matlab function sim_switch_vol_hover_rotation/Controlleur_hover_NL_rot/split ==
  data: f input; nu input; f_d output size=1; q_d input; q_r input; omega_d output size=3; controlleur parameter; err output
function [f_d, omega_d, err] = split(f, nu, q_d, q_r, controlleur)
%#codegen

R_d = q2dcm(q_d);

eta_d = q_d(1);
eps_d = q_d(2:4);

eta_r = q_r(1);
eps_r = q_r(2:4);

eps_delta_prime = -eta_d*eps_r + eta_r*eps_d - skew_sym(eps_r)*eps_d;

f_d = (R_d * controlleur.d_etoile)' * nu;
omega_d = 1/f * controlleur.skew_sym_d_etoile * R_d' * nu -controlleur.kq*controlleur.d_etoile*controlleur.d_etoile'*eps_delta_prime;

err =  R_d*controlleur.d_etoile*f_d + skew_sym(omega_d) * controlleur.d_etoile * f - nu;

== matlab function sim_switch_vol_hover_rotation/Controlleur_hover_NL_rot/f_delta stab ==
  data: f input; f_delta input; nu output; e input; q_omega input; q_d input; controlleur parameter; drone parameter
function nu = stab_f_delta(f, f_delta, e, q_omega, q_d, controlleur, drone)
%#codegen
m = drone.MASS;
kpp = controlleur.kpp;
kpd = controlleur.kpd;
k_delta = controlleur.k_delta;

ep = e(1:3);
ev = e(4:6);

q = q_omega(1:4);
% omega = q_omega(5:7);

R = q2dcm(q);
Rd = q2dcm(q_d);

nu = ((kpp * kpd)/m) * ep + (kpd^2/m - kpp) * ev - (kpd/m + k_delta) * f_delta -kpd/m * (R-Rd) * controlleur.d_etoile * f;

== matlab function sim_switch_vol_hover_rotation/MATLAB Function3 ==
  data: u input; y output
function y = fcn(u)
%#codegen

y = norm(u);

== matlab function sim_switch_vol_hover_rotation/Controlleur_hover_NL_rot/e stab ==
  data: e input; f_r output; drone parameter; controlleur parameter
function f_r = e_stab(e, drone, controlleur)
%#codegen
ep = e(1:3);
ev = e(4:6);

f_r = drone.MASS * [0;0;drone.G] - controlleur.kpp * ep - controlleur.kpd * ev;

== matlab function sim_switch_vol_hover_rotation/Controlleur_hover_NL_rot/feedforward ==
  data: f input; omega_dd output; q_d input; f_delta input; e input; q_omega input; omega_d input; nu input; controlleur parameter; drone parameter; omega_d1_p output; omega_d2_p output; omega_d3_p output
function [omega_dd, omega_d1_p, omega_d2_p, omega_d3_p]  = feedforward(f, q_d, f_delta,e, q_omega,omega_d, nu, controlleur, drone)
%#codegen

d_etoile = controlleur.d_etoile;
kpp = controlleur.kpp;
kpd = controlleur.kpd;
k_delta = controlleur.k_delta;
m = drone.MASS;

ep = e(1:3);
ev = e(4:6);

q = q_omega(1:4);
omega = q_omega(5:7);

R = q2dcm(q);
Rd = q2dcm(q_d);

omega_d1_p = -(1/(f^2)) * skew_sym(d_etoile) * Rd' * nu * ( Rd * d_etoile)' * nu;
omega_d2_p = -(1/(f))* skew_sym(d_etoile) * skew_sym(omega_d) * Rd' * nu;

Gain = (kpd^2/m^2 - kpp/m);

ep_term = - Gain*kpp*ep;
ev_term = (kpp*kpd/m - Gain*kpd)*ev;
f_delta_term = (Gain + (kpd/m + k_delta)*k_delta)*f_delta;
f_term = (Gain*(R-Rd) + kpd/m * (Rd*skew_sym(omega_d) - R*skew_sym(omega)))*d_etoile* f;
nu_term = kpd/m * (Rd-R) * d_etoile * (Rd*d_etoile)'* nu;

omega_d3_p = (1/f) * skew_sym(d_etoile) * Rd'* (ep_term + ev_term + f_delta_term + f_term + nu_term); 

omega_dd = omega_d1_p + omega_d2_p + omega_d3_p ; %
